simulink model "sensor_airgap"  (R2022b)
settings: Solver=VariableStepAuto  StartTime=0.0  StopTime=10.0  RelTol=1e-3
settings Model: Creator=aceao  LastModifiedBy=USUARIO

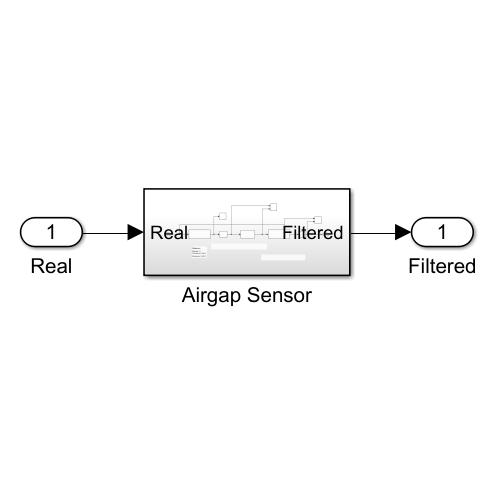
[thumbnail: Simulink's stored preview of the top-level diagram]
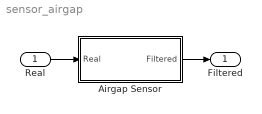
== system sensor_airgap ==
  Real : Inport
  Airgap Sensor : Subsystem
  Filtered : Outport
  wires:
  Real/1 -> Airgap Sensor/1(Real)
  Airgap Sensor/1(Filtered) -> Filtered/1

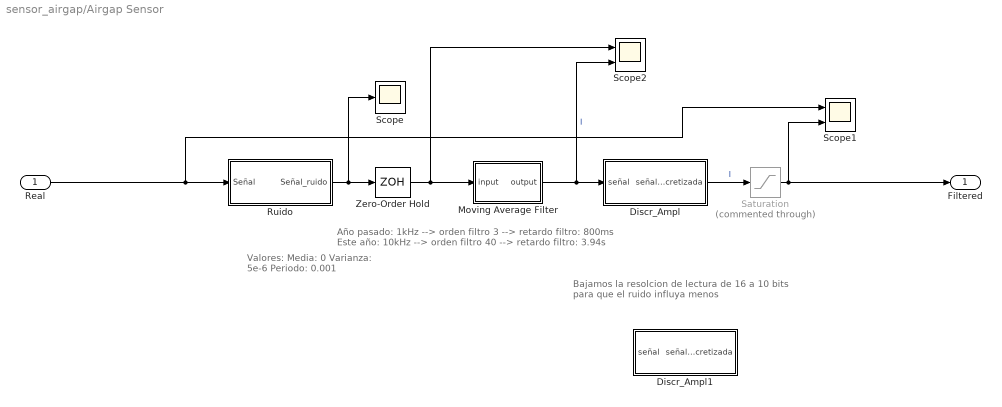
== system sensor_airgap/Airgap Sensor ==
  note: Bajamos la resolcion de lectura de 16 a 10 bits
      | para que el ruido influya menos
  note: Año pasado: 1kHz --> orden filtro 3 --> retardo filtro: 800ms
      | Este año: 10kHz --> orden filtro 40  --> retardo filtro: 3.94s
  note: Valores:
      | Media: 0
      | Varianza: 5e-6
      | Periodo: 0.001
  Real : Inport
  Discr_Ampl : Subsystem  mask{N=2048, Min=0.045, Max=0.125}
      mask prompts: N "Valores distintos (N)"; Min "Valor mínimo"; Max "Valor máximo"
      mask DialogControl DescGroupVar Prompt: Discretizacion_Amplitud
      mask DialogControl DescTextVar Prompt: Discretización en amplitud
  Discr_Ampl1 : Subsystem  mask{N=1024, Min=0.065, Max=0.105}
      mask prompts: N "Valores distintos (N)"; Min "Valor mínimo"; Max "Valor máximo"
      mask DialogControl DescGroupVar Prompt: Discretizacion_Amplitud
      mask DialogControl DescTextVar Prompt: Discretización en amplitud
  Moving Average Filter : Subsystem  mask{M=40, fs=-1}
      mask prompts: M "Orden del filtro (M)"; fs "Frecuencia de muestreo (fs)"
  Ruido : Subsystem  mask{M=0, V=5e-8, T=0.00001}
      mask prompts: M "Media"; V "Varianza"; T "Periodo"
      mask DialogControl Ruido Prompt: Ruido
      mask DialogControl DescTextVar Prompt: Añade ruido gaussiano
  Saturation : Saturate  Commented=through  UpperLimit=0.105  LowerLimit=0.065
  Scope : Scope
  Scope1 : Scope  NumInputPorts=2
  Scope2 : Scope  NumInputPorts=2
  Zero-Order Hold : ZeroOrderHold  SampleTime=1/(10*10^3)
  Filtered : Outport
  wires:
  Real/1 -> Scope1/1, Ruido/1(Señal)
  Discr_Ampl/1(señal_discretizada) -> Saturation/1  "I"
  Moving Average Filter/1(output) -> Discr_Ampl/1(señal), Scope2/2  "I"
  Ruido/1(Señal_ruido) -> Scope/1, Zero-Order Hold/1
  Zero-Order Hold/1 -> Moving Average Filter/1(input), Scope2/1
  Saturation/1 -> Filtered/1, Scope1/2

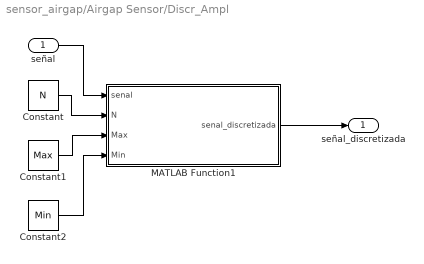
== system sensor_airgap/Airgap Sensor/Discr_Ampl ==
  señal : Inport
  Constant : Constant  Value=N
  Constant1 : Constant  Value=Max
  Constant2 : Constant  Value=Min
  MATLAB Function1 : MATLAB Function  TreatAsAtomicUnit=on
  señal_discretizada : Outport
  wires:
  MATLAB Function1/1(senal_discretizada) -> señal_discretizada/1
  señal/1 -> MATLAB Function1/1(senal)
  Constant1/1 -> MATLAB Function1/3(Max)
  Constant/1 -> MATLAB Function1/2(N)
  Constant2/1 -> MATLAB Function1/4(Min)

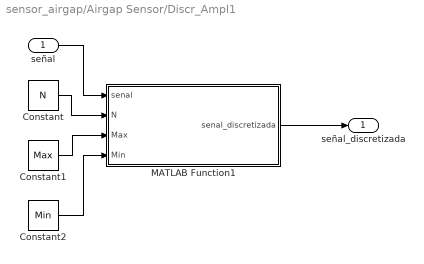
== system sensor_airgap/Airgap Sensor/Discr_Ampl1 ==
  señal : Inport
  Constant : Constant  Value=N
  Constant1 : Constant  Value=Max
  Constant2 : Constant  Value=Min
  MATLAB Function1 : MATLAB Function  TreatAsAtomicUnit=on
  señal_discretizada : Outport
  wires:
  MATLAB Function1/1(senal_discretizada) -> señal_discretizada/1
  señal/1 -> MATLAB Function1/1(senal)
  Constant1/1 -> MATLAB Function1/3(Max)
  Constant/1 -> MATLAB Function1/2(N)
  Constant2/1 -> MATLAB Function1/4(Min)

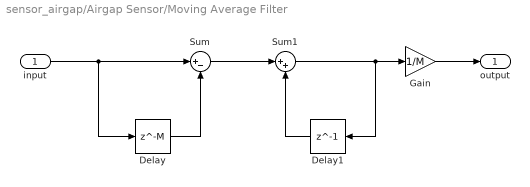
== system sensor_airgap/Airgap Sensor/Moving Average Filter ==
  input : Inport
  Delay : Delay  DelayLength=M  SampleTime=fs
  Delay1 : Delay  DelayLength=1  SampleTime=fs
  Gain : Gain  Gain=1/M
  Sum : Sum  Inputs=|+-
  Sum1 : Sum  Inputs=|++
  output : Outport
  wires:
  input/1 -> Delay/1, Sum/1
  Delay/1 -> Sum/2
  Sum/1 -> Sum1/1
  Sum1/1 -> Delay1/1, Gain/1
  Delay1/1 -> Sum1/2
  Gain/1 -> output/1

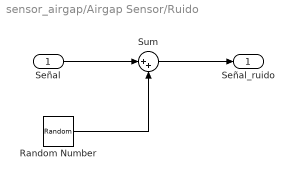
== system sensor_airgap/Airgap Sensor/Ruido ==
  Señal : Inport
  Random Number : RandomNumber  Mean=M  Variance=V  Seed=3  SampleTime=T
  Sum : Sum  Inputs=|++
  Señal_ruido : Outport
  wires:
  Random Number/1 -> Sum/2
  Señal/1 -> Sum/1
  Sum/1 -> Señal_ruido/1

== matlab function sensor_airgap/Airgap Sensor/Discr_Ampl1/MATLAB Function1 ==
  data: senal input; senal_discretizada output; N input; Max input; Min input
function senal_discretizada  = fcn(senal,N,Max,Min)

if(senal>Max)
    senal_discretizada=Max;
    return
elseif(senal<Min)
    senal_discretizada=Min;
    return
end

valor_escalon=(Max-Min)/(N-1);
i=Min;
 while(i<Max)
    if(i+valor_escalon/2>senal)
        senal_discretizada=i;
        return
    end
    i=i+valor_escalon;
end

      senal_discretizada=Max;
end

== matlab function sensor_airgap/Airgap Sensor/Discr_Ampl/MATLAB Function1 ==
  data: senal input; senal_discretizada output; N input; Max input; Min input
function senal_discretizada  = fcn(senal,N,Max,Min)

if(senal>Max)
    senal_discretizada=Max;
    return
elseif(senal<Min)
    senal_discretizada=Min;
    return
end

valor_escalon=(Max-Min)/(N-1);
i=Min;
 while(i<Max)
    if(i+valor_escalon/2>senal)
        senal_discretizada=i;
        return
    end
    i=i+valor_escalon;
end

      senal_discretizada=Max;
end
